simulink library "lib_Serial_Realtime"  (R2018b)
settings: Solver=VariableStepAuto  StartTime=0.0  StopTime=10.0  RelTol=1e-3
undefined symbols (not defined in the file or in its folder): ipaddr, macaddr, PTP, Standard_Devices, UDP_Protocol
libraries: ptplib x17, xpcutilitieslib x4, xpcethernetlib x4, sldrtlib x2, xpcrtudplib x2
settings Model: xpc_rtwmakecfg_data=_xpciplib__xpcetherlib__xpcether8255xlib__xpcetherGbElib_  Creator=m.hiepp  LastModifiedBy=m.hiepp

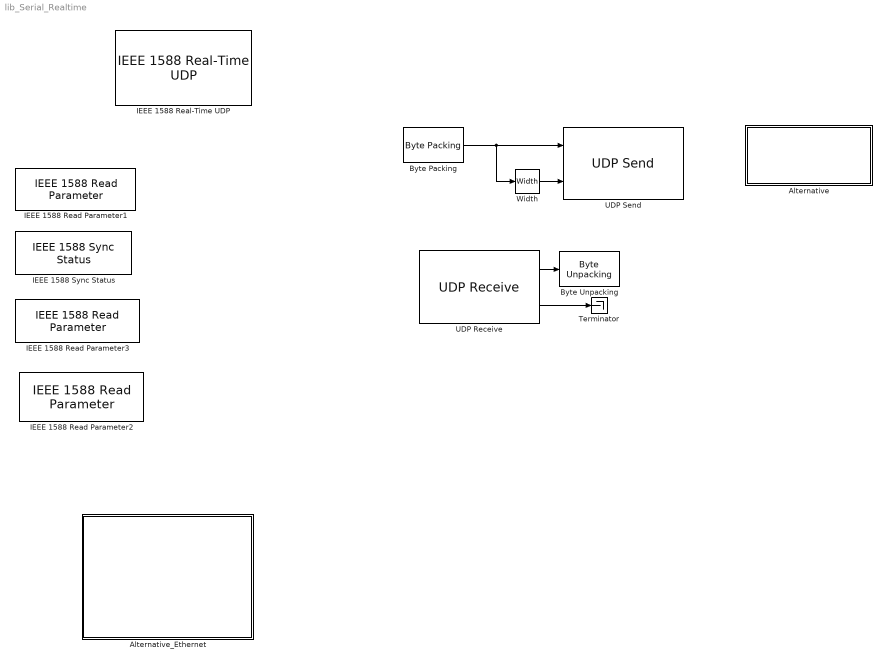
== system lib_Serial_Realtime ==
  Alternative : Subsystem
  Alternative_Ethernet : Subsystem
  "Byte Packing " : xpcutilitieslib/Byte Packing   MaskPackedDataType=uint8  MaskUnpackedDataTypes={'double'}  MaskAlignment=1
  "Byte Unpacking " : xpcutilitieslib/Byte Unpacking   MaskUnpackedDataTypes={'double'}  MaskUnpackedDataSizes={[1]}  MaskAlignment=1
      settings: SourceProductName=Simulink Real-Time  SourceProductBaseCode=XP
  IEEE 1588 Read Parameter1 : ptplib/IEEE 1588 Read Parameter  Priority=1  ID=1  param=Protocol state  sample_time=0.01  enable_read_precision=off
      settings: SourceProductName=Simulink Real-Time  SourceProductBaseCode=XP
  IEEE 1588 Read Parameter2 : ptplib/IEEE 1588 Read Parameter  Priority=1  ID=1  param=Offset from Master  sample_time=0.01  enable_read_precision=off
      settings: SourceProductName=Simulink Real-Time  SourceProductBaseCode=XP
  IEEE 1588 Read Parameter3 : ptplib/IEEE 1588 Read Parameter  Priority=1  ID=1  param=PTP time (time-of-day)  sample_time=0.01  enable_read_precision=off
      settings: SourceProductName=Simulink Real-Time  SourceProductBaseCode=XP
  IEEE 1588 Sync Status : ptplib/IEEE 1588 Sync Status  Priority=1  ID=1  offset_threshold=10e-6  sample_time=0.01
      settings: SourceProductName=Simulink Real-Time  SourceProductBaseCode=XP
  IEEE 1588 Real-Time UDP : ptplib/IEEE 1588 Real-Time UDP  Priority=0  ID=1  PciBus=1  PciSlot=0  PciFunction=0  time_inc=4000000  sample_time=0.01  IpSource=Specify  IpAddress=30.30.30.1  SubnetMask=255.255.255.0  Gateway=0.0.0.0  Receive1=0.0.0.0  dest_ip_select=Standard PTP multicast (224.0.1.129, 224.0.0.107)  custom_dest_ip_addr=255.255.255.255  MulticastList=[ipaddr('224.0.1.129'), ipaddr('224.0.0.107')]  Multicast={macaddr('01:00:5E:00:01:81'), macaddr('01:00:5E:00:00:6B')}  time_source=Ethernet board  timescale=PTP (1970-01-01)  epoch=[1970 01 01 00]  delay_measure=Request-response  slave_only=off  enable_advanced_config=off  domain_num=0  utc_offset=35  priority1=128  clock_class=248  clock_accuracy=hex2dec('FE')  priority2=128  announce_interval=2  sync_interval=0.1  min_pdelay_req_interval=0.1  announce_receipt_timeout=3
      settings: SourceProductName=Simulink Real-Time  SourceProductBaseCode=XP
  Terminator : Terminator
  UDP Receive : xpcrtudplib/UDP Receive  ipAddressVal=Use host-target connection  localPort=8000  rcvWidth=8  rcvFmAny=on  fmAddress=30.30.30.2  rcvMulticast=off  multicastAddress={}  maxUDPQueue=8  sampleTime=0.01
      settings: SourceProductName=Simulink Real-Time
  UDP Send : xpcrtudplib/UDP Send  ipAddressVal=30.30.30.1  localPort=-1  toAddress=255.255.255.255  toPort=8001  sampleTime=-1
      settings: SourceProductName=Simulink Real-Time  SourceProductBaseCode=XP
  Width : Width
  wires:
  "Byte Packing "/1 -> Width/1, UDP Send/1
  Width/1 -> UDP Send/2
  UDP Receive/1 -> "Byte Unpacking "/1
  UDP Receive/2 -> Terminator/1

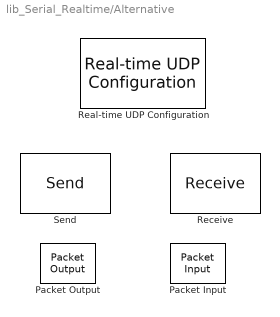
== system lib_Serial_Realtime/Alternative ==
  Packet Input : sldrtlib/Packet Input  SampleTime=0.01  MaxMissedTicks=50  ShowMissedTicks=off  YieldWhenWaiting=off  DrvName=Standard_Devices/UDP_Protocol  DrvAddress=36880  DrvOptions=[0 36864 108 111 99 97 108 104 111 115 116 0 0 0 0 0 0 0 0 0 0 0 0 0 0 0 0 0 0 0 0 0 0 0 0 0 0 0 0 0 0 0 0 0 0 0 0 0 0 0 0 0 0 0 0 0 0 0 0 0 0 0 0 0 0 0 0 0 0 0 0 0 0 0 0 0 0 0 0 0 0 0 0 0 0 0 0 0 0 0 0 0 0 0 0 0 0 0 0 0 0 0 0 0 0 0 0 0 0 0 0 0 0 0 0 0 0 0 0 0 0 0 0 0 0 0 0 0 0 0 0 0 0 0 0 0 0 0 0 0 0 0 0 0 0 0 0 0 0 0 0 0 0 0 0 0 0 0 0 0 0 0 0 0 0 0 0 0 0 0 0 0 0 0 0 0 0 0 0 0 0 0 0 0 0 0 0 0 0 0 0 0 0 0 0 0 0 0 0 0 0 0 0 0 0 0 0 0 0 0 0 0 0 0 0 0 0 0 0 0 0 0 0 0 0 0 0 0 0 0 0 0 0 0 0 0 0 0 0 0 0 0 0 0 0 0 0 0 0 0 0 0 0 0 0 0]  PacketSize=40  DataTypes={'4*double', '8*int8'}  ShowReady=off  ShowError=off  PacketID=1  ByteOrder=1  ShowTimestamp=off
      settings: AttributesFormatString=UDP Protocol [36880]  SourceProductName=Simulink Desktop Real-Time
  Packet Output : sldrtlib/Packet Output  SampleTime=0.01  MaxMissedTicks=50  ShowMissedTicks=off  YieldWhenWaiting=off  DrvName=Standard_Devices/UDP_Protocol  DrvAddress=36864  DrvOptions=[0 36880 108 111 99 97 108 104 111 115 116 0 0 0 0 0 0 0 0 0 0 0 0 0 0 0 0 0 0 0 0 0 0 0 0 0 0 0 0 0 0 0 0 0 0 0 0 0 0 0 0 0 0 0 0 0 0 0 0 0 0 0 0 0 0 0 0 0 0 0 0 0 0 0 0 0 0 0 0 0 0 0 0 0 0 0 0 0 0 0 0 0 0 0 0 0 0 0 0 0 0 0 0 0 0 0 0 0 0 0 0 0 0 0 0 0 0 0 0 0 0 0 0 0 0 0 0 0 0 0 0 0 0 0 0 0 0 0 0 0 0 0 0 0 0 0 0 0 0 0 0 0 0 0 0 0 0 0 0 0 0 0 0 0 0 0 0 0 0 0 0 0 0 0 0 0 0 0 0 0 0 0 0 0 0 0 0 0 0 0 0 0 0 0 0 0 0 0 0 0 0 0 0 0 0 0 0 0 0 0 0 0 0 0 0 0 0 0 0 0 0 0 0 0 0 0 0 0 0 0 0 0 0 0 0 0 0 0 0 0 0 0 0 0 0 0 0 0 0 0 0 0 0 0 0 0]  PacketSize=40  DataTypes={'4*double', '8*int8'}  ShowReady=off  ShowError=off  PacketID=1  ByteOrder=1  InitialValue=[]  FinalValue=[]
      settings: AttributesFormatString=UDP Protocol [36864]  SourceProductName=Simulink Desktop Real-Time
  "Real-time UDP Configuration " : ptplib/PTP UDP/Real-time UDP  Configuration   ID=1  IpAddress=0.0.0.0  SubnetMask=255.255.255.0  Gateway=0.0.0.0  EthDrv=Intel 8255x  PciBus=[]  PciSlot=[]  PciFunction=0  udpID=0  MulticastList=[]  Multicast={}
      settings: SourceProductName=Simulink Real-Time  SourceProductBaseCode=XP
  "Receive " : ptplib/PTP UDP/Receive   ID=1  Receive1=0.0.0.0  Receive2=25000  Receive3=1  Receive4=-1  udpID=0
      settings: SourceProductName=Simulink Real-Time  SourceProductBaseCode=XP
  "Send " : ptplib/PTP UDP/Send   ID=1  Send1=255.255.255.255  Send2=25000  Send3=-1  Send4=-1  udpID=0
      settings: SourceProductName=Simulink Real-Time  SourceProductBaseCode=XP

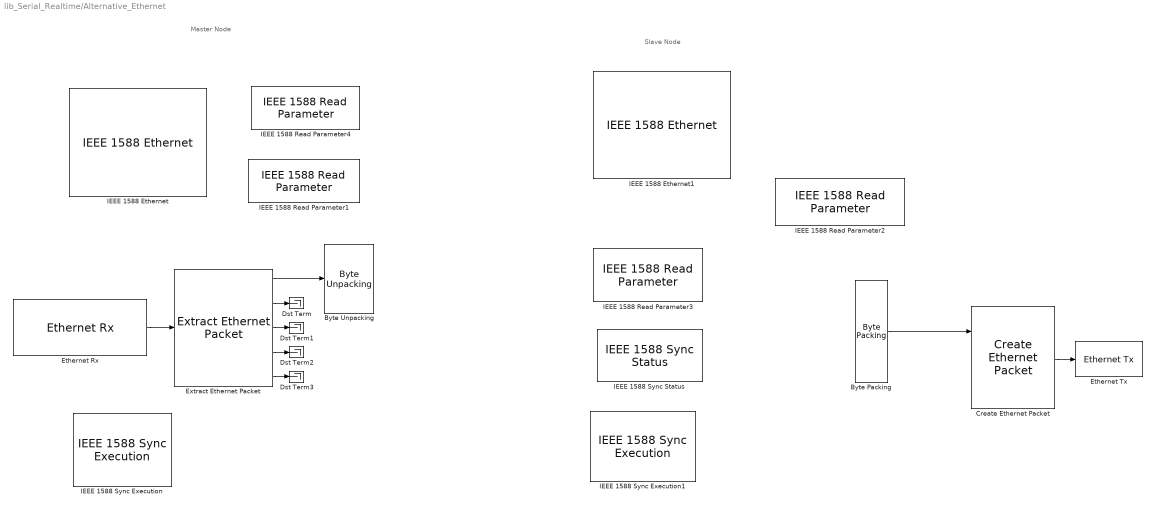
== system lib_Serial_Realtime/Alternative_Ethernet ==
  note: Slave Node
  note: Master Node
  "Byte Packing " : xpcutilitieslib/Byte Packing   MaskPackedDataType=uint8  MaskUnpackedDataTypes={'uint8', 'double', 'double'}  MaskAlignment=1
  "Byte Unpacking " : xpcutilitieslib/Byte Unpacking   MaskUnpackedDataTypes={'uint8','double','double'}  MaskUnpackedDataSizes={1,1,1}  MaskAlignment=1
      settings: SourceProductName=Simulink Real-Time  SourceProductBaseCode=XP
  "Create Ethernet Packet " : xpcethernetlib/Create Ethernet Packet   DstMac=macaddr('50:50:50:50:50:50')  EtherType=17
      settings: SourceProductName=Simulink Real-Time  SourceProductBaseCode=XP
  Dst Term{,1..3} (4 alike) : Terminator
  "Ethernet Rx " : xpcethernetlib/Ethernet Rx   ID=1  SampleTime=0.01  Criteria=Specify types to match  EtherType=[17]  BlkID=0
      settings: SourceProductName=Simulink Real-Time  SourceProductBaseCode=XP
  "Ethernet Tx " : xpcethernetlib/Ethernet Tx   ID=1  SampleTime=0.01
      settings: SourceProductName=Simulink Real-Time  SourceProductBaseCode=XP
  "Extract Ethernet Packet " : xpcethernetlib/Extract Ethernet Packet   EthernetDataSize=17
      settings: SourceProductName=Simulink Real-Time  SourceProductBaseCode=XP
  IEEE 1588 Read Parameter1 : ptplib/IEEE 1588 Read Parameter  ID=1  param=PTP time (time-of-day)  sample_time=0.01  enable_read_precision=off
      settings: SourceProductName=Simulink Real-Time  SourceProductBaseCode=XP
  IEEE 1588 Read Parameter2 : ptplib/IEEE 1588 Read Parameter  ID=1  param=Offset from Master  sample_time=0.01  enable_read_precision=off
      settings: SourceProductName=Simulink Real-Time  SourceProductBaseCode=XP
  IEEE 1588 Read Parameter3 : ptplib/IEEE 1588 Read Parameter  ID=1  param=Protocol state  sample_time=0.01  enable_read_precision=off
      settings: SourceProductName=Simulink Real-Time  SourceProductBaseCode=XP
  IEEE 1588 Read Parameter4 : ptplib/IEEE 1588 Read Parameter  ID=1  param=Protocol state  sample_time=0.01  enable_read_precision=off
      settings: SourceProductName=Simulink Real-Time  SourceProductBaseCode=XP
  IEEE 1588 Sync Status : ptplib/IEEE 1588 Sync Status  ID=1  offset_threshold=1e-6  sample_time=0.01
      settings: SourceProductName=Simulink Real-Time  SourceProductBaseCode=XP
  IEEE 1588 Ethernet : ptplib/IEEE 1588 Ethernet  Priority=0  ID=1  PciBus=5  PciSlot=0  PciFunction=0  time_inc=4000000  sample_time=0.01  AddressSource=Specify  MAC=macaddr('50:50:50:50:50:50')  mac_select=Standard PTP multicast (01:1B:19:00:00:00, 01:80:C2:00:00:0E)  dest_mac=00:00:00:00:00:00  time_source=Ethernet board  timescale=PTP (1970-01-01)  epoch=[1970 01 01 00]  delay_measure=Request-response  slave_only=off  enable_advanced_config=off  domain_num=0  utc_offset=35  priority1=128  clock_class=248  clock_accuracy=hex2dec('FE')  priority2=128  announce_interval=2  sync_interval=0.1  min_pdelay_req_interval=0.1  announce_receipt_timeout=3
      settings: SourceProductName=Simulink Real-Time  SourceProductBaseCode=XP
  IEEE 1588 Ethernet1 : ptplib/IEEE 1588 Ethernet  Priority=0  ID=1  PciBus=5  PciSlot=0  PciFunction=0  time_inc=4000000  sample_time=0.01  AddressSource=EEPROM  MAC=macaddr('00:00:00:00:00:00')  mac_select=Standard PTP multicast (01:1B:19:00:00:00, 01:80:C2:00:00:0E)  dest_mac=00:00:00:00:00:00  time_source=Ethernet board  timescale=PTP (1970-01-01)  epoch=[1970 01 01 00]  delay_measure=Request-response  slave_only=on  enable_advanced_config=off  domain_num=0  utc_offset=35  priority1=128  clock_class=248  clock_accuracy=hex2dec('FE')  priority2=128  announce_interval=2  sync_interval=0.1  min_pdelay_req_interval=0.1  announce_receipt_timeout=3
      settings: SourceProductName=Simulink Real-Time  SourceProductBaseCode=XP
  IEEE 1588 Sync Execution : ptplib/IEEE 1588 Sync Execution  Gain=.1  PoleZ=0.7  offset_threshold=1e-3  sample_time=0.01
      settings: SourceProductName=Simulink Real-Time  SourceProductBaseCode=XP
  IEEE 1588 Sync Execution1 : ptplib/IEEE 1588 Sync Execution  Gain=0.1  PoleZ=0.7  offset_threshold=1e-3  sample_time=0.01
      settings: SourceProductName=Simulink Real-Time  SourceProductBaseCode=XP
  wires:
  "Extract Ethernet Packet "/2 -> Dst Term/1
  "Extract Ethernet Packet "/1 -> "Byte Unpacking "/1
  "Extract Ethernet Packet "/3 -> Dst Term1/1
  "Extract Ethernet Packet "/5 -> Dst Term3/1
  "Ethernet Rx "/1 -> "Extract Ethernet Packet "/1
  "Extract Ethernet Packet "/4 -> Dst Term2/1
  "Byte Packing "/1 -> "Create Ethernet Packet "/1
  "Create Ethernet Packet "/1 -> "Ethernet Tx "/1
